simulink model "lift_flowchart"  (R2020b)
settings: Solver=VariableStepAuto  StartTime=0.0  StopTime=10.0  RelTol=1e-3
settings Model: Creator=DELL  LastModifiedBy=DELL

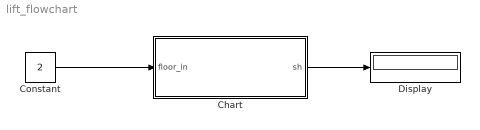
== system lift_flowchart ==
  Chart : Stateflow chart  TreatAsAtomicUnit=on
  Constant : Constant  Value=2
  Display : Display
  wires:
  Constant/1 -> Chart/1(floor_in)
  Chart/1(sh) -> Display/1

== stateflow chart lift_flowchart/Chart ==
  (default) -> (junction 1) : {curr_st=0;}
  (junction 11) -> (junction 1) [order 1] : [curr_st~=floor_in]
  (junction 1) -> (junction 3) [order 1] : [curr_st<=floor_in]
  (junction 1) -> (junction 8) [order 2]
  (junction 3) -> (junction 5) : {curr_st=curr_st+1;}
  (junction 8) -> (junction 9) [order 1] : [curr_st>=floor_in]
  (junction 8) -> (junction 11) [order 2] : {curr_st=0;}
  (junction 9) -> (junction 10) : {curr_st=curr_st-1;}
  (junction 10) -> (junction 11)
  (junction 5) -> (junction 10)
  (junction 11) -> (junction 12) [order 2] : {sh=curr_st;}
  data: curr_st local =0; sh output; floor_in input
